simulink model "RegressFil_CodeGen_Interper_Different_Result"  (R2017b)
settings: Solver=VariableStepAuto  StartTime=0.0  StopTime=10.0  RelTol=1e-3
settings Model: Creator=81068  LastModifiedBy=81068

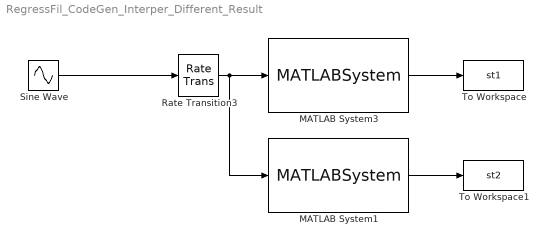
== system RegressFil_CodeGen_Interper_Different_Result ==
  MATLAB System1 : MATLABSystem  System=PolyRegressionFilter  sample_time=sample_time  history_length=history_length  dop=15  signal_dim=1  SimulateUsing=Interpreted execution
      mask Type: PolyRegressionFilter
      mask Display:
      | disp('PolyRegressionFilter');
      | port_label('input',1,'q');
      | port_label('output',1,'dq');
  MATLAB System3 : MATLABSystem  System=PolyRegressionFilter  sample_time=sample_time  history_length=history_length  dop=15  signal_dim=1  SimulateUsing=Code generation
      mask Type: PolyRegressionFilter
      mask Display:
      | disp('PolyRegressionFilter');
      | port_label('input',1,'q');
      | port_label('output',1,'dq');
  Rate Transition3 : RateTransition  OutPortSampleTime=1/2000
  Sine Wave : Sin  SampleTime=0
  To Workspace : ToWorkspace  VariableName=st1  SaveFormat=Timeseries  SampleTime=-1
  To Workspace1 : ToWorkspace  VariableName=st2  SaveFormat=Timeseries  SampleTime=-1
  wires:
  Sine Wave/1 -> Rate Transition3/1
  MATLAB System3/1 -> To Workspace/1
  MATLAB System1/1 -> To Workspace1/1
  Rate Transition3/1 -> MATLAB System1/1, MATLAB System3/1
